simulink model "Autopilot_q_full_5may_new"  (R2020a)
settings: Solver=ode4  StartTime=0.0  StopTime=300  FixedStep=0.01  RelTol=1e-3
undefined symbols (not defined in the file or in its folder): Aero_cofficients, Atmosphere_pert, Atmospheric_model, Counter_sensor_model, Earth, error_global, flags_global, Guidance_Flags_global, INT_global, param_guidance, Payload_data, Plane_state_mode_finish_catcher_ftr_mode, Plane_state_mode_finish_catcher_fw_mode, Plane_state_mode_finish_catcher_q_mode, Plane_state_mode_finish_catcher_rtr_mode, Plane_state_store, propulsion_model, propulsion_model_int, Structural_data, Thrust_data_store, time_global, WGS84, Wind_data, Wind_model_int, Wind_pert_factor
libraries: simulink x33, aerolibactuator x15, cstblocks x3, aerolibatmos2 x2, aerolibfltsims x1, aerolibtransform2 x1, shared6dof x1
(part 6 of 10)

== system Autopilot_q_full_5may_new/AUTOPILOT /Autopilot Transition mode/Reverse transition/Pitch Controller/alpha controller ==
  acc_d : Inport
  Plane_state : Inport  Port=2
  Action Port : ActionPort  ActionPortLabel=else { }
  Aero_coffecients read2 : DataStoreRead  DataStoreName=Aero_cofficients  DataStoreElements=Aero_cofficients(:,:)
  Constant{6..11} (6 alike) : Constant
  Data Store Read : DataStoreRead  DataStoreName=Thrust_data_store  DataStoreElements=Thrust_data_store(:,:)
  Data Store Read1 : DataStoreRead  DataStoreName=Wind_data  DataStoreElements=Wind_data(:)
  Data Store Read13 : DataStoreRead  DataStoreName=propulsion_model  DataStoreElements=propulsion_model(:)
  Data Store Read15 : DataStoreRead  DataStoreName=Atmospheric_model
  Gain : Gain  Gain=57.3
  Gain1 : Gain  Gain=57.3
  MATLAB Function3 : MATLAB Function  TreatAsAtomicUnit=on
  PID Controller (2DOF)2 : simulink/Continuous/PID Controller (2DOF)  Controller=PID  TimeDomain=Discrete-time  SampleTime=0.01  IntegratorMethod=Forward Euler  FilterMethod=Forward Euler  Form=Parallel  UseFilter=on  ControllerParametersSource=internal  P=4.0  I=0.3  D=0.0  N=100  b=1  c=1  InitialConditionSource=internal  InitialConditionForIntegrator=0  InitialConditionForFilter=0  ExternalReset=none  ZeroCross=off  LimitOutput=off  UpperSaturationLimit=inf  LowerSaturationLimit=-inf  LinearizeAsGain=on  AntiWindupMode=none  Kb=1  TrackingMode=off  Kt=1  PParamMin=[]  PParamMax=[]  IParamMin=[]  IParamMax=[]  DParamMin=[]  DParamMax=[]  NParamMin=[]  NParamMax=[]  bParamMin=[]  bParamMax=[]  cParamMin=[]  cParamMax=[]  KbParamMin=[]  KbParamMax=[]  KtParamMin=[]  KtParamMax=[]  POutMin=[]  POutMax=[]  IOutMin=[]  IOutMax=[]  DOutMin=[]  DOutMax=[]  NOutMin=[]  NOutMax=[]  bOutMin=[]  bOutMax=[]  cOutMin=[]  cOutMax=[]  KbOutMin=[]  KbOutMax=[]  KtOutMin=[]  KtOutMax=[]  IntegratorOutMin=[]  IntegratorOutMax=[]  FilterOutMin=[]  FilterOutMax=[]  SumOutMin=[]  SumOutMax=[]  Sum1OutMin=[]  Sum1OutMax=[]  Sum2OutMin=[]  Sum2OutMax=[]  Sum3OutMin=[]  Sum3OutMax=[]  SumI1OutMin=[]  SumI1OutMax=[]  SumI2OutMin=[]  SumI2OutMax=[]  SumI3OutMin=[]  SumI3OutMax=[]  SumDOutMin=[]  SumDOutMax=[]  SaturationOutMin=[]  SaturationOutMax=[]  IntegratorContinuousStateAttributes=''  IntegratorStateMustResolveToSignalObject=off  IntegratorRTWStateStorageClass=Auto  FilterContinuousStateAttributes=''  FilterStateMustResolveToSignalObject=off  FilterRTWStateStorageClass=Auto  DifferentiatorICPrevScaledInput=0  DifferentiatorOutMin=[]  DifferentiatorOutMax=[]  FilterDiffOutCoefMin=[]  FilterDiffOutCoefMax=[]  SumDenOutMin=[]  SumDenOutMax=[]  SumNumOutMin=[]  SumNumOutMax=[]  ReciprocalOutMin=[]  ReciprocalOutMax=[]  DivideOutMin=[]  DivideOutMax=[]  TunerSelectOption=Transfer Function Based (PID Tuner App)
  Scope : Scope  NumInputPorts=2
  Structure_data_read1 : DataStoreRead  DataStoreName=Structural_data  DataStoreElements=Structural_data(:,:)
  alpha : Trigonometry  Operator=atan2
  u : DataStoreRead  DataStoreName=Plane_state_store  DataStoreElements=Plane_state_store(1,1)
  w : DataStoreRead  DataStoreName=Plane_state_store  DataStoreElements=Plane_state_store(1,3)
  Output : Outport  VectorParamsAs1DForOutWhenUnconnected=off
  wires:
  PID Controller (2DOF)2/1 -> Output/1
  Plane_state/1 -> MATLAB Function3/2(Plane_state)
  acc_d/1 -> MATLAB Function3/1(acc_d)
  MATLAB Function3/1(alpha_d) -> Gain/1, PID Controller (2DOF)2/1
  w/1 -> alpha/1
  u/1 -> alpha/2
  alpha/1 -> Gain1/1, PID Controller (2DOF)2/2
  Data Store Read/1 -> MATLAB Function3/5(Thrust)
  Aero_coffecients read2/1 -> MATLAB Function3/3(aero_data)
  Structure_data_read1/1 -> MATLAB Function3/4(structure_data)
  Gain1/1 -> Scope/2
  Gain/1 -> Scope/1
  Data Store Read1/1 -> MATLAB Function3/6(Wind_ned)
  Data Store Read13/1 -> MATLAB Function3/7(propulsion_data)
  Data Store Read15/1 -> MATLAB Function3/8(atmos_data)
  Constant6/1 -> MATLAB Function3/9(data2)
  Constant7/1 -> MATLAB Function3/10(data3)
  Constant8/1 -> MATLAB Function3/11(data4)
  Constant9/1 -> MATLAB Function3/12(data5)
  Constant10/1 -> MATLAB Function3/13(data6)
  Constant11/1 -> MATLAB Function3/14(data7)

== system Autopilot_q_full_5may_new/AUTOPILOT /Autopilot Transition mode/Reverse transition/Pitch Controller/theta controller ==
  time : Inport
  a_x_d : Inport  Port=2
  alpha_trim : Inport  Port=3
  Action Port : ActionPort  ActionPortLabel=if { }
  Data Store Read1 : DataStoreRead  DataStoreName=Thrust_data_store  DataStoreElements=Thrust_data_store(1,1:8)
  Gain : Gain  Gain=57.3
  Gain1 : Gain  Gain=57.3
  MATLAB Function3 : MATLAB Function  TreatAsAtomicUnit=on
  PID Controller (2DOF)2 : simulink/Continuous/PID Controller (2DOF)  Controller=PID  TimeDomain=Discrete-time  SampleTime=0.01  IntegratorMethod=Forward Euler  FilterMethod=Forward Euler  Form=Parallel  UseFilter=on  ControllerParametersSource=internal  P=2.0  I=0.0  D=0  N=100  b=1  c=1  InitialConditionSource=internal  InitialConditionForIntegrator=0  InitialConditionForFilter=0  ExternalReset=none  LimitOutput=off  UpperSaturationLimit=inf  LowerSaturationLimit=-inf  LinearizeAsGain=on  AntiWindupMode=none  Kb=1  TrackingMode=off  Kt=1  PParamMin=[]  PParamMax=[]  IParamMin=[]  IParamMax=[]  DParamMin=[]  DParamMax=[]  NParamMin=[]  NParamMax=[]  bParamMin=[]  bParamMax=[]  cParamMin=[]  cParamMax=[]  KbParamMin=[]  KbParamMax=[]  KtParamMin=[]  KtParamMax=[]  POutMin=[]  POutMax=[]  IOutMin=[]  IOutMax=[]  DOutMin=[]  DOutMax=[]  NOutMin=[]  NOutMax=[]  bOutMin=[]  bOutMax=[]  cOutMin=[]  cOutMax=[]  KbOutMin=[]  KbOutMax=[]  KtOutMin=[]  KtOutMax=[]  IntegratorOutMin=[]  IntegratorOutMax=[]  FilterOutMin=[]  FilterOutMax=[]  SumOutMin=[]  SumOutMax=[]  Sum1OutMin=[]  Sum1OutMax=[]  Sum2OutMin=[]  Sum2OutMax=[]  Sum3OutMin=[]  Sum3OutMax=[]  SumI1OutMin=[]  SumI1OutMax=[]  SumI2OutMin=[]  SumI2OutMax=[]  SumI3OutMin=[]  SumI3OutMax=[]  SumDOutMin=[]  SumDOutMax=[]  SaturationOutMin=[]  SaturationOutMax=[]  IntegratorContinuousStateAttributes=''  IntegratorStateMustResolveToSignalObject=off  IntegratorRTWStateStorageClass=Auto  FilterContinuousStateAttributes=''  FilterStateMustResolveToSignalObject=off  FilterRTWStateStorageClass=Auto  DifferentiatorICPrevScaledInput=0  DifferentiatorOutMin=[]  DifferentiatorOutMax=[]  FilterDiffOutCoefMin=[]  FilterDiffOutCoefMax=[]  SumDenOutMin=[]  SumDenOutMax=[]  SumNumOutMin=[]  SumNumOutMax=[]  ReciprocalOutMin=[]  ReciprocalOutMax=[]  DivideOutMin=[]  DivideOutMax=[]  TunerSelectOption=Transfer Function Based (PID Tuner App)
  Scope : Scope  NumInputPorts=2
  mass : DataStoreRead  DataStoreName=Structural_data  DataStoreElements=Structural_data(1,1)
  theta : DataStoreRead  DataStoreName=Plane_state_store  DataStoreElements=Plane_state_store(1,8)
  theta_dot : Outport  VectorParamsAs1DForOutWhenUnconnected=off
  wires:
  theta/1 -> PID Controller (2DOF)2/2, Gain1/1
  time/1 -> MATLAB Function3/1(t)
  Data Store Read1/1 -> MATLAB Function3/2(TT)
  a_x_d/1 -> MATLAB Function3/4(a_x_d)
  PID Controller (2DOF)2/1 -> theta_dot/1
  alpha_trim/1 -> MATLAB Function3/5(data)
  mass/1 -> MATLAB Function3/3(mass)
  MATLAB Function3/1(theta_d) -> Gain/1, PID Controller (2DOF)2/1
  Gain1/1 -> Scope/2
  Gain/1 -> Scope/1

== system Autopilot_q_full_5may_new/INITIALISE_PARAMS/If Action Subsystem/Aero_data_perturbation/Subsystem1/Subsystem ==
  CL_alpha : Constant
  CL_beta : Constant
  CL_delta_a : Constant
  CL_delta_e : Constant
  CL_delta_r : Constant
  CLo : Constant
  CLp : Constant
  CLq : Constant
  CLr : Constant
  Mux : Mux  Inputs=9
  Out1 : Outport  VectorParamsAs1DForOutWhenUnconnected=off
  wires:
  CL_delta_e/1 -> Mux/4
  CL_delta_r/1 -> Mux/6
  CLp/1 -> Mux/7
  CLo/1 -> Mux/1
  CL_alpha/1 -> Mux/2
  CLr/1 -> Mux/9
  CL_delta_a/1 -> Mux/5
  CL_beta/1 -> Mux/3
  CLq/1 -> Mux/8
  Mux/1 -> Out1/1

== system Autopilot_q_full_5may_new/INITIALISE_PARAMS/If Action Subsystem/Aero_data_perturbation/Subsystem2/Subsystem ==
  CL_alpha : Constant
  CL_beta : Constant
  CL_delta_a : Constant
  CL_delta_e : Constant
  CL_delta_r : Constant
  CLo : Constant
  CLp : Constant
  CLq : Constant
  CLr : Constant
  Mux : Mux  Inputs=9
  Out1 : Outport  VectorParamsAs1DForOutWhenUnconnected=off
  wires:
  Mux/1 -> Out1/1
  CLq/1 -> Mux/8
  CL_beta/1 -> Mux/3
  CL_delta_a/1 -> Mux/5
  CLr/1 -> Mux/9
  CL_alpha/1 -> Mux/2
  CLo/1 -> Mux/1
  CLp/1 -> Mux/7
  CL_delta_r/1 -> Mux/6
  CL_delta_e/1 -> Mux/4

== system Autopilot_q_full_5may_new/INITIALISE_PARAMS/If Action Subsystem/Aero_data_perturbation/Subsystem3/Subsystem ==
  CL_alpha : Constant
  CL_beta : Constant
  CL_delta_a : Constant
  CL_delta_e : Constant
  CL_delta_r : Constant
  CLo : Constant
  CLp : Constant
  CLq : Constant
  CLr : Constant
  Mux : Mux  Inputs=9
  Out1 : Outport  VectorParamsAs1DForOutWhenUnconnected=off
  wires:
  CL_delta_e/1 -> Mux/4
  CL_delta_r/1 -> Mux/6
  CLp/1 -> Mux/7
  CLo/1 -> Mux/1
  CL_alpha/1 -> Mux/2
  CLr/1 -> Mux/9
  CL_delta_a/1 -> Mux/5
  CL_beta/1 -> Mux/3
  CLq/1 -> Mux/8
  Mux/1 -> Out1/1

== system Autopilot_q_full_5may_new/INITIALISE_PARAMS/If Action Subsystem/Aero_data_perturbation/Subsystem4/Subsystem ==
  CL_alpha : Constant
  CL_beta : Constant
  CL_delta_a : Constant
  CL_delta_e : Constant
  CL_delta_r : Constant
  CLo : Constant
  CLp : Constant
  CLq : Constant
  CLr : Constant
  Mux : Mux  Inputs=9
  Out1 : Outport  VectorParamsAs1DForOutWhenUnconnected=off
  wires:
  Mux/1 -> Out1/1
  CLq/1 -> Mux/8
  CL_beta/1 -> Mux/3
  CL_delta_a/1 -> Mux/5
  CLr/1 -> Mux/9
  CL_alpha/1 -> Mux/2
  CLo/1 -> Mux/1
  CLp/1 -> Mux/7
  CL_delta_r/1 -> Mux/6
  CL_delta_e/1 -> Mux/4

== system Autopilot_q_full_5may_new/INITIALISE_PARAMS/If Action Subsystem/Aero_data_perturbation/Subsystem5/Subsystem ==
  CL_alpha : Constant
  CL_beta : Constant
  CL_delta_a : Constant
  CL_delta_e : Constant
  CL_delta_r : Constant
  CLo : Constant
  CLp : Constant
  CLq : Constant
  CLr : Constant
  Mux : Mux  Inputs=9
  Out1 : Outport  VectorParamsAs1DForOutWhenUnconnected=off
  wires:
  CL_delta_e/1 -> Mux/4
  CL_delta_r/1 -> Mux/6
  CLp/1 -> Mux/7
  CLo/1 -> Mux/1
  CL_alpha/1 -> Mux/2
  CLr/1 -> Mux/9
  CL_delta_a/1 -> Mux/5
  CL_beta/1 -> Mux/3
  CLq/1 -> Mux/8
  Mux/1 -> Out1/1

== system Autopilot_q_full_5may_new/INITIALISE_PARAMS/If Action Subsystem/Aero_data_perturbation/Subsystem6/Subsystem ==
  CL_alpha : Constant
  CL_beta : Constant
  CL_delta_a : Constant
  CL_delta_e : Constant
  CL_delta_r : Constant
  CLo : Constant
  CLp : Constant
  CLq : Constant
  CLr : Constant
  Mux : Mux  Inputs=9
  Out1 : Outport  VectorParamsAs1DForOutWhenUnconnected=off
  wires:
  Mux/1 -> Out1/1
  CLq/1 -> Mux/8
  CL_beta/1 -> Mux/3
  CL_delta_a/1 -> Mux/5
  CLr/1 -> Mux/9
  CL_alpha/1 -> Mux/2
  CLo/1 -> Mux/1
  CLp/1 -> Mux/7
  CL_delta_r/1 -> Mux/6
  CL_delta_e/1 -> Mux/4

== system Autopilot_q_full_5may_new/INITIALISE_PARAMS/If Action Subsystem/Atmosphere_pert/Subsystem1/Subsystem ==
  note: p
  note: density
  note: Temp
  note: a
  Constant{,1..3} (4 alike) : Constant
  Mux : Mux
  Out1 : Outport  VectorParamsAs1DForOutWhenUnconnected=off
  wires:
  Constant2/1 -> Mux/3
  Constant1/1 -> Mux/2
  Constant/1 -> Mux/1
  Constant3/1 -> Mux/4
  Mux/1 -> Out1/1

== system Autopilot_q_full_5may_new/INITIALISE_PARAMS/If Action Subsystem/Propulsion_data_pert/Subsystem1/Subsystem ==
  note: d_vtol
  note: b_vtol
  Constant : Constant
  Constant1 : Constant
  Mux : Mux  Inputs=2
  Out1 : Outport  VectorParamsAs1DForOutWhenUnconnected=off
  wires:
  Constant1/1 -> Mux/2
  Mux/1 -> Out1/1
  Constant/1 -> Mux/1

== system Autopilot_q_full_5may_new/INITIALISE_PARAMS/If Action Subsystem/Propulsion_data_pert/Subsystem2/Subsystem ==
  note: d_pusher
  note: b_pusher
  Constant2 : Constant
  Constant3 : Constant
  Mux1 : Mux  Inputs=2
  Out1 : Outport  VectorParamsAs1DForOutWhenUnconnected=off
  wires:
  Mux1/1 -> Out1/1
  Constant3/1 -> Mux1/2
  Constant2/1 -> Mux1/1

== system Autopilot_q_full_5may_new/INITIALISE_PARAMS/If Action Subsystem/Structure_data_pert/Subsystem1/Subsystem ==
  Constant : Constant
  Out1 : Outport  VectorParamsAs1DForOutWhenUnconnected=off
  wires:
  Constant/1 -> Out1/1

== system Autopilot_q_full_5may_new/INITIALISE_PARAMS/If Action Subsystem/Structure_data_pert/Subsystem2/Subsystem ==
  Constant : Constant
  Constant1 : Constant
  Constant2 : Constant
  Mux : Mux  Inputs=3
  Out1 : Outport  VectorParamsAs1DForOutWhenUnconnected=off
  wires:
  Constant/1 -> Mux/1
  Mux/1 -> Out1/1
  Constant1/1 -> Mux/2
  Constant2/1 -> Mux/3

== system Autopilot_q_full_5may_new/INITIALISE_PARAMS/If Action Subsystem/Structure_data_pert/Subsystem3/Subsystem ==
  Constant{3..8} (6 alike) : Constant
  Mux1 : Mux  Inputs=6
  Out1 : Outport  VectorParamsAs1DForOutWhenUnconnected=off
  wires:
  Constant8/1 -> Mux1/6
  Mux1/1 -> Out1/1
  Constant3/1 -> Mux1/1
  Constant7/1 -> Mux1/5
  Constant5/1 -> Mux1/3
  Constant4/1 -> Mux1/2
  Constant6/1 -> Mux1/4

== system Autopilot_q_full_5may_new/INITIALISE_PARAMS/If Action Subsystem/Structure_data_pert/Subsystem4/Subsystem ==
  note: y9
  note: z1
  note: y10
  note: y5
  note: y7
  note: y6
  note: x2 y
  note: y2
  note: x1
  note: y8
  note: y4
  note: y1
  note: y3
  Constant{9..21} (13 alike) : Constant
  Mux2 : Mux  Inputs=13
  Out1 : Outport  VectorParamsAs1DForOutWhenUnconnected=off
  wires:
  Constant20/1 -> Mux2/7
  Constant17/1 -> Mux2/10
  Constant15/1 -> Mux2/8
  Constant19/1 -> Mux2/12
  Constant21/1 -> Mux2/13
  Constant12/1 -> Mux2/4
  Constant11/1 -> Mux2/3
  Mux2/1 -> Out1/1
  Constant10/1 -> Mux2/2
  Constant18/1 -> Mux2/11
  Constant14/1 -> Mux2/6
  Constant13/1 -> Mux2/5
  Constant16/1 -> Mux2/9
  Constant9/1 -> Mux2/1

== system Autopilot_q_full_5may_new/INITIALISE_PARAMS/If Action Subsystem/Structure_data_pert/Subsystem5/Subsystem ==
  mb_pert : Constant
  Out1 : Outport  VectorParamsAs1DForOutWhenUnconnected=off
  wires:
  mb_pert/1 -> Out1/1

== system Autopilot_q_full_5may_new/INITIALISE_PARAMS/If Action Subsystem/Wind_data_pert/Subsystem1/Subsystem ==
  note: V_N
  note: V_D
  note: V_E
  Constant : Constant
  Constant1 : Constant
  Constant2 : Constant
  Mux : Mux  Inputs=3
  Out1 : Outport  VectorParamsAs1DForOutWhenUnconnected=off
  wires:
  Constant/1 -> Mux/1
  Mux/1 -> Out1/1
  Constant1/1 -> Mux/2
  Constant2/1 -> Mux/3

== matlab function Autopilot_q_full_5may_new/All SENSOR MODEL2/MATLAB Function1 ==
  settings: updateMethod=DISCRETE
  data: sigma input; mu input; y output
function y = fcn(sigma,mu)
y=normrnd(mu,sigma);
end

== matlab function Autopilot_q_full_5may_new/All SENSOR MODEL2/MATLAB Function10 ==
  settings: updateMethod=DISCRETE
  data: sigma input; mu input; y output
function y = fcn(sigma,mu)
y=normrnd(mu,sigma);
end

== matlab function Autopilot_q_full_5may_new/All SENSOR MODEL2/MATLAB Function11 ==
  settings: updateMethod=DISCRETE
  data: sigma input; mu input; y output
function y = fcn(sigma,mu)
y=normrnd(mu,sigma);
end

== matlab function Autopilot_q_full_5may_new/All SENSOR MODEL2/MATLAB Function2 ==
  data: sigma input; mu input; y output
function y = fcn(sigma,mu)
y=normrnd(mu,sigma);
end

== matlab function Autopilot_q_full_5may_new/All SENSOR MODEL2/MATLAB Function3 ==
  data: sigma input; mu input; y output
function y = fcn(sigma,mu)
y=normrnd(mu,sigma);
end

== matlab function Autopilot_q_full_5may_new/All SENSOR MODEL2/MATLAB Function4 ==
  data: sigma input; mu input; y output
function y = fcn(sigma,mu)
y=normrnd(mu,sigma);
end

== matlab function Autopilot_q_full_5may_new/All SENSOR MODEL2/MATLAB Function5 ==
  data: sigma input; mu input; y output
function y = fcn(sigma,mu)
y=normrnd(mu,sigma);
end

== matlab function Autopilot_q_full_5may_new/All SENSOR MODEL2/MATLAB Function6 ==
  data: sigma input; mu input; y output
function y = fcn(sigma,mu)
y=normrnd(mu,sigma);
end

== matlab function Autopilot_q_full_5may_new/All SENSOR MODEL2/MATLAB Function7 ==
  data: sigma input; mu input; y output
function y = fcn(sigma,mu)
y=normrnd(mu,sigma);
end

== matlab function Autopilot_q_full_5may_new/All SENSOR MODEL2/MATLAB Function8 ==
  data: sigma input; mu input; y output
function y = fcn(sigma,mu)
y=normrnd(mu,sigma);
end

== matlab function Autopilot_q_full_5may_new/AUTOPILOT /Autopilot Transition mode/Reverse transition/Pitch Controller/MATLAB Function ==
  data: u1 input; u2 input; y output
function y = fcn(u1, u2)

if u1<u2    
    y=1; 
else
    y=0;
end


end

== matlab function Autopilot_q_full_5may_new/Wind_Model/Subsystem2/MATLAB Function ==
  data: u input; y output; Wind_model_int input; Z input
function y = fcn(u, Wind_model_int, Z)
y=u;
turb_50=Wind_model_int(8);
turb_50_600=Wind_model_int(9);
turb_600=Wind_model_int(10);

if ((turb_50 == 0) && (Z >=-50))
    y=0.0;  
end

if ((turb_50_600 == 0) && (Z >=-600) && (Z <=-50))
    y=0.0;  
end

if ((turb_600 == 0) && (Z <=-600))
    y=0.0;  
end

if Z>0.0
    y=0.0;
end
end

== matlab function Autopilot_q_full_5may_new/Forces and moments/Forces and moments ==
  data: Tzf1 input; Tzf2 input; Tzf3 input; Tzf4 input; Tzb5 input; Tzb6 input; Tzb7 input; Tzb8 input; Tx9 input; Tx10 input; delta_e input; delta_a input; delta_r input; fx output; fy output; fz output; l output; m output; n output; aero_data input; structure_data input; ideal_Plane_state input; Payload_f_m input; Wind_ned input; flags_global input; propulsion_data input; atmos_data input; wind_pert_factor input; propulsion_pert_factor input; structure_pert_factor input; atmos_pert_factor input; aero_coff_pert_factor input; data7 input; data8 input; data9 input; data10 input; data11 input; data12 input
function [fx,fy,fz,l,m,n] = fcn(Tzf1,Tzf2,Tzf3,Tzf4,Tzb5,Tzb6,Tzb7,Tzb8,Tx9,Tx10,delta_e,delta_a,delta_r, aero_data,structure_data , ideal_Plane_state, Payload_f_m,Wind_ned, flags_global, propulsion_data, atmos_data, wind_pert_factor, propulsion_pert_factor, structure_pert_factor, atmos_pert_factor, aero_coff_pert_factor, data7, data8, data9, data10, data11, data12)


quad_mode=flags_global(3);
Transition_mode=flags_global(4);
Fixed_wing_mode=flags_global(5);

%%
b1=propulsion_data(1); % b and d of vtol propellers
d1=propulsion_data(2);

b1 = b1*propulsion_pert_factor(1); % adding in perturbation in b and d
d1 = d1*propulsion_pert_factor(2);
b1_inv=1.0/b1;
%%
rho=atmos_data(4); % density
rho = rho*atmos_pert_factor(4); % adding perturbation in density
%%
mass=structure_data(1,1);c=structure_data(1,2);b=structure_data(1,3);s=structure_data(1,4);
Ix=structure_data(1,5);Iy=structure_data(1,6);Iz=structure_data(1,7);
Ixy=structure_data(1,8);Ixz=structure_data(1,9);Iyz=structure_data(1,10);
x1=structure_data(1,11);x2=structure_data(1,12);y1=structure_data(1,13);y2=structure_data(1,14);
y3=structure_data(1,15);y4=structure_data(1,16);y5=structure_data(1,17);y6=structure_data(1,18);
y7=structure_data(1,19);y8=structure_data(1,20);y9=structure_data(1,21);y10=structure_data(1,22);
z9=structure_data(1,23);mb=structure_data(1,24);
%%
mass=mass*structure_pert_factor(1,1); % perturbation in structure data
c=c*structure_pert_factor(1,2);b=b*structure_pert_factor(1,3);s=s*structure_pert_factor(1,4);
Ix=Ix*structure_pert_factor(1,5);Iy=Iy*structure_pert_factor(1,6);Iz=Iz*structure_pert_factor(1,7);
Ixy=Ixy*structure_pert_factor(1,8);Ixz=Ixz*structure_pert_factor(1,9);Iyz=Iyz*structure_pert_factor(1,10);
x1=x1*structure_pert_factor(1,11);x2=x2*structure_pert_factor(1,12);
y1=y1*structure_pert_factor(1,13);y2=y2*structure_pert_factor(1,14);y3=y3*structure_pert_factor(1,15);y4=y4*structure_pert_factor(1,16);
y5=y5*structure_pert_factor(1,17);y6=y6*structure_pert_factor(1,18);y7=y7*structure_pert_factor(1,19);y8=y8*structure_pert_factor(1,20);
y9=y9*structure_pert_factor(1,21);y10=y10*structure_pert_factor(1,22);
z9=z9*structure_pert_factor(1,23);
mb=mb*structure_pert_factor(1,24);
z10=-z9;
%%
c0=Ix*Iz-Ixz^2;
c1=Ixz*(Ix-Iy+Iz)/c0;
c2=(Iz*(Iz-Iy)+Ixz^2)/c0;
c3=Iz/c0;
c4=Ixz/c0;
c5=(Iz-Ix)/c0;
c6=Ixz/Iy;
c7=((Ix-Iy)*Ix + Ixz^2)/c0;
c8=Ix/c0;
%%

CLo =aero_data(1,1); CL_alpha=aero_data(1,2);CL_beta=aero_data(1,3); CL_delta_e=aero_data(1,4); CL_delta_a=aero_data(1,5); CL_delta_r=aero_data(1,6); CL_p=aero_data(1,7);CL_q=aero_data(1,8);CL_r=aero_data(1,9);

Cdo =aero_data(2,1); Cd_alpha=aero_data(2,2);Cd_beta=aero_data(2,3); Cd_delta_e=aero_data(2,4); Cd_delta_a=aero_data(2,5); Cd_delta_r=aero_data(2,6); Cd_p=aero_data(2,7);Cd_q=aero_data(2,8);Cd_r=aero_data(2,9);

CYo =aero_data(3,1); CY_alpha=aero_data(3,2);CY_beta=aero_data(3,3); CY_delta_e=aero_data(3,4); CY_delta_a=aero_data(3,5); CY_delta_r=aero_data(3,6); CY_p=aero_data(3,7);CY_q=aero_data(3,8);CY_r=aero_data(3,9);

Clo =aero_data(4,1); Cl_alpha=aero_data(4,2);Cl_beta=aero_data(4,3); Cl_delta_e=aero_data(4,4); Cl_delta_a=aero_data(4,5); Cl_delta_r=aero_data(4,6); Cl_p=aero_data(4,7);Cl_q=aero_data(4,8);Cl_r=aero_data(4,9);

Cmo =aero_data(5,1); Cm_alpha=aero_data(5,2);Cm_beta=aero_data(5,3); Cm_delta_e=aero_data(5,4); Cm_delta_a=aero_data(5,5); Cm_delta_r=aero_data(5,6); Cm_p=aero_data(5,7);Cm_q=aero_data(5,8);Cm_r=aero_data(5,9);

Cno =aero_data(6,1); Cn_alpha=aero_data(6,2);Cn_beta=aero_data(6,3); Cn_delta_e=aero_data(6,4); Cn_delta_a=aero_data(6,5); Cn_delta_r=aero_data(6,6); Cn_p=aero_data(6,7);Cn_q=aero_data(6,8);Cn_r=aero_data(6,9);

if quad_mode ==1
    aero_data(:,:)=0.0;
    CLo =aero_data(1,1); CL_alpha=aero_data(1,2);CL_beta=aero_data(1,3); CL_delta_e=aero_data(1,4); CL_delta_a=aero_data(1,5); CL_delta_r=aero_data(1,6); CL_p=aero_data(1,7);CL_q=aero_data(1,8);CL_r=aero_data(1,9);
    
    Cdo =aero_data(2,1); Cd_alpha=aero_data(2,2);Cd_beta=aero_data(2,3); Cd_delta_e=aero_data(2,4); Cd_delta_a=aero_data(2,5); Cd_delta_r=aero_data(2,6); Cd_p=aero_data(2,7);Cd_q=aero_data(2,8);Cd_r=aero_data(2,9);
    
    CYo =aero_data(3,1); CY_alpha=aero_data(3,2);CY_beta=aero_data(3,3); CY_delta_e=aero_data(3,4); CY_delta_a=aero_data(3,5); CY_delta_r=aero_data(3,6); CY_p=aero_data(3,7);CY_q=aero_data(3,8);CY_r=aero_data(3,9);
    
    Clo =aero_data(4,1); Cl_alpha=aero_data(4,2);Cl_beta=aero_data(4,3); Cl_delta_e=aero_data(4,4); Cl_delta_a=aero_data(4,5); Cl_delta_r=aero_data(4,6); Cl_p=aero_data(4,7);Cl_q=aero_data(4,8);Cl_r=aero_data(4,9);
    
    Cmo =aero_data(5,1); Cm_alpha=aero_data(5,2);Cm_beta=aero_data(5,3); Cm_delta_e=aero_data(5,4); Cm_delta_a=aero_data(5,5); Cm_delta_r=aero_data(5,6); Cm_p=aero_data(5,7);Cm_q=aero_data(5,8);Cm_r=aero_data(5,9);
    
    Cno =aero_data(6,1); Cn_alpha=aero_data(6,2);Cn_beta=aero_data(6,3); Cn_delta_e=aero_data(6,4); Cn_delta_a=aero_data(6,5); Cn_delta_r=aero_data(6,6); Cn_p=aero_data(6,7);Cn_q=aero_data(6,8);Cn_r=aero_data(6,9);
end

if Fixed_wing_mode ==1
    
    CLo =aero_data(1,1); CL_alpha=aero_data(1,2);CL_beta=aero_data(1,3); CL_delta_e=aero_data(1,4); CL_delta_a=aero_data(1,5); CL_delta_r=aero_data(1,6); CL_p=aero_data(1,7);CL_q=aero_data(1,8);CL_r=aero_data(1,9);
    
    Cdo =aero_data(2,1); Cd_alpha=aero_data(2,2);Cd_beta=aero_data(2,3); Cd_delta_e=aero_data(2,4); Cd_delta_a=aero_data(2,5); Cd_delta_r=aero_data(2,6); Cd_p=aero_data(2,7);Cd_q=aero_data(2,8);Cd_r=aero_data(2,9);
    
    CYo =aero_data(3,1); CY_alpha=aero_data(3,2);CY_beta=aero_data(3,3); CY_delta_e=aero_data(3,4); CY_delta_a=aero_data(3,5); CY_delta_r=aero_data(3,6); CY_p=aero_data(3,7);CY_q=aero_data(3,8);CY_r=aero_data(3,9);
    
    Clo =aero_data(4,1); Cl_alpha=aero_data(4,2);Cl_beta=aero_data(4,3); Cl_delta_e=aero_data(4,4); Cl_delta_a=aero_data(4,5); Cl_delta_r=aero_data(4,6); Cl_p=aero_data(4,7);Cl_q=aero_data(4,8);Cl_r=aero_data(4,9);
    
    Cmo =aero_data(5,1); Cm_alpha=aero_data(5,2);Cm_beta=aero_data(5,3); Cm_delta_e=aero_data(5,4); Cm_delta_a=aero_data(5,5); Cm_delta_r=aero_data(5,6); Cm_p=aero_data(5,7);Cm_q=aero_data(5,8);Cm_r=aero_data(5,9);
    
    Cno =aero_data(6,1); Cn_alpha=aero_data(6,2);Cn_beta=aero_data(6,3); Cn_delta_e=aero_data(6,4); Cn_delta_a=aero_data(6,5); Cn_delta_r=aero_data(6,6); Cn_p=aero_data(6,7);Cn_q=aero_data(6,8);Cn_r=aero_data(6,9);
end

if Transition_mode==1
    CLo =aero_data(1,1); CL_alpha=aero_data(1,2);CL_beta=aero_data(1,3); CL_delta_e=aero_data(1,4); CL_delta_a=aero_data(1,5); CL_delta_r=aero_data(1,6); CL_p=aero_data(1,7);CL_q=aero_data(1,8);CL_r=aero_data(1,9);
    
    Cdo =aero_data(2,1); Cd_alpha=aero_data(2,2);Cd_beta=aero_data(2,3); Cd_delta_e=aero_data(2,4); Cd_delta_a=aero_data(2,5); Cd_delta_r=aero_data(2,6); Cd_p=aero_data(2,7);Cd_q=aero_data(2,8);Cd_r=aero_data(2,9);
    
    CYo =aero_data(3,1); CY_alpha=aero_data(3,2);CY_beta=aero_data(3,3); CY_delta_e=aero_data(3,4); CY_delta_a=aero_data(3,5); CY_delta_r=aero_data(3,6); CY_p=aero_data(3,7);CY_q=aero_data(3,8);CY_r=aero_data(3,9);
    
    Clo =aero_data(4,1); Cl_alpha=aero_data(4,2);Cl_beta=aero_data(4,3); Cl_delta_e=aero_data(4,4); Cl_delta_a=aero_data(4,5); Cl_delta_r=aero_data(4,6); Cl_p=aero_data(4,7);Cl_q=aero_data(4,8);Cl_r=aero_data(4,9);
    
    Cmo =aero_data(5,1); Cm_alpha=aero_data(5,2);Cm_beta=aero_data(5,3); Cm_delta_e=aero_data(5,4); Cm_delta_a=aero_data(5,5); Cm_delta_r=aero_data(5,6); Cm_p=aero_data(5,7);Cm_q=aero_data(5,8);Cm_r=aero_data(5,9);
    
    Cno =aero_data(6,1); Cn_alpha=aero_data(6,2);Cn_beta=aero_data(6,3); Cn_delta_e=aero_data(6,4); Cn_delta_a=aero_data(6,5); Cn_delta_r=aero_data(6,6); Cn_p=aero_data(6,7);Cn_q=aero_data(6,8);Cn_r=aero_data(6,9);
end
%% perturbation in Aero coffecients
CLo =CLo*aero_coff_pert_factor(1,1); CL_alpha=CL_alpha*aero_coff_pert_factor(1,2);CL_beta=CL_beta*aero_coff_pert_factor(1,3); CL_delta_e=CL_delta_e*aero_coff_pert_factor(1,4); CL_delta_a=CL_delta_a*aero_coff_pert_factor(1,5); CL_delta_r=CL_delta_r*aero_coff_pert_factor(1,6); CL_p=CL_p*aero_coff_pert_factor(1,7);CL_q=CL_q*aero_coff_pert_factor(1,8);CL_r=CL_r*aero_coff_pert_factor(1,9);

Cdo =Cdo*aero_coff_pert_factor(2,1); Cd_alpha=Cd_alpha*aero_coff_pert_factor(2,2);Cd_beta=Cd_beta*aero_coff_pert_factor(2,3); Cd_delta_e=Cd_delta_e*aero_coff_pert_factor(2,4); Cd_delta_a=Cd_delta_a*aero_coff_pert_factor(2,5); Cd_delta_r=Cd_delta_r*aero_coff_pert_factor(2,6); Cd_p=Cd_p*aero_coff_pert_factor(2,7);Cd_q=Cd_q*aero_coff_pert_factor(2,8);Cd_r=Cd_r*aero_coff_pert_factor(2,9);

CYo =CYo*aero_coff_pert_factor(3,1); CY_alpha=CY_alpha*aero_coff_pert_factor(3,2);CY_beta=CY_beta*aero_coff_pert_factor(3,3); CY_delta_e=CY_delta_e*aero_coff_pert_factor(3,4); CY_delta_a=CY_delta_a*aero_coff_pert_factor(3,5); CY_delta_r=CY_delta_r*aero_coff_pert_factor(3,6); CY_p=CY_p*aero_coff_pert_factor(3,7);CY_q=CY_q*aero_coff_pert_factor(3,8);CY_r=CY_r*aero_coff_pert_factor(3,9);

Clo =Clo*aero_coff_pert_factor(4,1); Cl_alpha=Cl_alpha*aero_coff_pert_factor(4,2);Cl_beta=Cl_beta*aero_coff_pert_factor(4,3); Cl_delta_e=Cl_delta_e*aero_coff_pert_factor(4,4); Cl_delta_a=Cl_delta_a*aero_coff_pert_factor(4,5); Cl_delta_r=Cl_delta_r*aero_coff_pert_factor(4,6); Cl_p=Cl_p*aero_coff_pert_factor(4,7);Cl_q=Cl_q*aero_coff_pert_factor(4,8);Cl_r=Cl_r*aero_coff_pert_factor(4,9);

Cmo =Cmo*aero_coff_pert_factor(5,1); Cm_alpha=Cm_alpha*aero_coff_pert_factor(5,2);Cm_beta=Cm_beta*aero_coff_pert_factor(5,3); Cm_delta_e=Cm_delta_e*aero_coff_pert_factor(5,4); Cm_delta_a=Cm_delta_a*aero_coff_pert_factor(5,5); Cm_delta_r=Cm_delta_r*aero_coff_pert_factor(5,6); Cm_p=Cm_p*aero_coff_pert_factor(5,7);Cm_q=Cm_q*aero_coff_pert_factor(5,8);Cm_r=Cm_r*aero_coff_pert_factor(5,9);

Cno =Cno*aero_coff_pert_factor(6,1); Cn_alpha=Cn_alpha*aero_coff_pert_factor(6,2);Cn_beta=Cn_beta*aero_coff_pert_factor(6,3); Cn_delta_e=Cn_delta_e*aero_coff_pert_factor(6,4); Cn_delta_a=Cn_delta_a*aero_coff_pert_factor(6,5); Cn_delta_r=Cn_delta_r*aero_coff_pert_factor(6,6); Cn_p=Cn_p*aero_coff_pert_factor(6,7);Cn_q=Cn_q*aero_coff_pert_factor(6,8);Cn_r=Cn_r*aero_coff_pert_factor(6,9);
%%
Cd_brake=0.0;brake=0.0;g=9.81;
%%
u=ideal_Plane_state(1);
v=ideal_Plane_state(2);
w=ideal_Plane_state(3);
p=ideal_Plane_state(4);
q=ideal_Plane_state(5);
r=ideal_Plane_state(6);
phi=ideal_Plane_state(7);
theta=ideal_Plane_state(8);
psi=ideal_Plane_state(9);
X=ideal_Plane_state(10);
Y=ideal_Plane_state(11);
Z=ideal_Plane_state(12);
%%


Tzf=Tzf2+Tzf3;
Tzb=Tzb6+Tzb7;
%%

R_v_v1=[cos(psi) sin(psi) 0; -sin(psi) cos(psi) 0; 0 0 1];
R_v1_v2=[cos(theta) 0 -sin(theta) ;0 1 0; sin(theta) 0 cos(theta)];
R_v2_b=[1 0 0;0 cos(phi) sin(phi) ;0 -sin(phi) cos(phi)];
R_v_b=R_v2_b*R_v1_v2*R_v_v1;

%%

Wind_ned(1)=Wind_ned(1)*wind_pert_factor(1);% adding perturbation to wind components
Wind_ned(2)=Wind_ned(2)*wind_pert_factor(2);
Wind_ned(3)=Wind_ned(3)*wind_pert_factor(3);

V_wind_bd=R_v_b*[Wind_ned(1);Wind_ned(2);Wind_ned(3)];

ppp = [u-V_wind_bd(1); v-V_wind_bd(2); w-V_wind_bd(3)];
u_r=ppp(1);
v_r=ppp(2);
w_r=ppp(3);
V=sqrt(u_r^2+v_r^2+w_r^2);

%%

if (u_r^2+v_r^2+w_r^2)<=0.01
    alpha=0;
else
    alpha=atan2( w_r, u_r);
end


if norm(u_r) < 10^-3  && norm(v_r) < 10^-3 && norm(w_r) < 10^-3
    beta=0;
else
    beta = asin(v_r/sqrt(u_r^2+v_r^2+w_r^2));
end
%%


R_b_s=[cos(alpha) 0 sin(alpha) ;0 1 0; -sin(alpha) 0 cos(alpha)];
R_s_w=[cos(beta) sin(beta) 0; -sin(beta) cos(beta) 0; 0 0 1];
R_w_b=(R_b_s)'*(R_s_w)';

%%


mg_b = R_v_b*[0 ;0; mass*g];
D=0.5*rho*V*V*s*(Cdo+Cd_alpha*abs(alpha)+Cd_delta_e*abs(delta_e)+ Cd_brake*abs(brake)) ;
D_b=R_w_b*[-D;0;0];

if V<0.1
    CL = CLo + CL_alpha*alpha + CL_delta_e*delta_e ;
else
    CL = CLo + CL_alpha*alpha + CL_delta_e*delta_e  + CL_q*q*c/(2*V) ;
end
L=0.5*rho*V*V*s*(CL);
L_b = R_w_b*[0;0;-L];
if abs(V)<0.1
    CY=CYo + CY_delta_r*delta_r + CY_beta*beta;
else
    CY=CYo + CY_delta_r*delta_r + CY_beta*beta + CY_r*r*b/(2*V);
end
FY=0.5*rho*V*V*s*(CY);
%%

l_aero=0.5*rho*V^2*s*b*( Clo + Cl_delta_a*delta_a +Cl_delta_r*delta_r +Cl_beta*beta )+0.5*rho*V*s*b*(Cl_p*p*b/2+Cl_r*r*b/2);
m_aero=0.5*rho*V^2*s*c*( Cmo + Cm_alpha*alpha + Cm_delta_e*delta_e)+0.5*rho*V*s*c*Cm_q*q*c/2;
n_aero=0.5*rho*V^2*s*b*( Cno + Cn_delta_a*delta_a +Cn_delta_r*delta_r +Cn_beta*beta )+0.5*rho*V*s*b*(Cn_r*r*b/2+ Cn_p*p*b/2);


l=Payload_f_m(3) + l_aero - Tzf2*y2*cos(mb) - Tzf3*y3*cos(mb)   - Tzb6*y6*cos(mb) - Tzb7*y7*cos(mb);
m=Payload_f_m(4) + m_aero + Tzf*x1*cos(mb) + Tzb*x2*cos(mb) + Tx9*z9 + d1*Tzf2*b1_inv*sin(mb) - d1*Tzf3*b1_inv*sin(mb) - d1*Tzb6*b1_inv*sin(mb) + d1*Tzb7*b1_inv*sin(mb) ;
%n=n_aero - Tx9_real*y9  - d1*Tzf2_real/b1 + d1*Tzf3_real/b1 + d1*Tzb6_real/b1 - d1*Tzb7_real/b1 ; //optimization
n=Payload_f_m(5) + n_aero - Tx9*y9 - Tx10*y10 + (Tzf2*x1*sin(mb) - Tzf3*x1*sin(mb) +  Tzb6*x2*sin(mb) - Tzb7*x2*sin(mb)) - d1*Tzf2*b1_inv*cos(mb) + d1*Tzf3*b1_inv*cos(mb)  + d1*Tzb6*b1_inv*cos(mb)  - d1*Tzb7*b1_inv*cos(mb)  ;



fx = Payload_f_m(1) +  Tx9 + Tx10 + D_b(1)+ mg_b(1)+L_b(1);
%%%%%%%%%%%%%%%%%%%%%%%%%%%%%%%%%%%%%%%%%%%%%%%%%%%%%%%%%%%%%%%%%%%%%%%%%%%
fy = Payload_f_m(2) + (Tzf2*sin(mb) - Tzf3*sin(mb) + Tzb6*sin(mb) - Tzb7*sin(mb)) + D_b(2) + mg_b(2) + FY + L_b(2);
%%%%%%%%%%%%%%%%%%%%%%%%%%%%%%%%%%%%%%%%%%%%%%%%%%%%%%%%%%%%%%%%%%%%%%%%%%%
fz = Payload_f_m(3) -  Tzf*cos(mb) - Tzb*cos(mb) + mg_b(3)+D_b(3)+L_b(3);



end

== matlab function Autopilot_q_full_5may_new/All SENSOR MODEL2/MATLAB Function9 ==
  data: sigma input; mu input; y output
function y = fcn(sigma,mu)
y=normrnd(mu,sigma);
end

== matlab function Autopilot_q_full_5may_new/AUTOPILOT /Autopilot Quad mode/Autopilot ==
  data: q_dot_d input; p_dot_d input; r_dot_d input; acc_d input; Tzf1 output; Tzf2 output; Tzf3 output; Tzf4 output; Tzb5 output; Tzb6 output; Tzb7 output; Tzb8 output; Tx9 output; Tx10 output; delta_e output; delta_a output; delta_r output; Plane_state input; aero_data input; structure_data input; Thrust input; Wind_ned input; propulsion_data input; atmos_data input; wind_pert_factor input; propulsion_pert_factor input; structure_pert_factor input; atmos_pert_factor input; aero_coff_pert_factor input; data7 input; data8 input; data9 input; data10 input; data11 input; data12 input
function [Tzf1,Tzf2,Tzf3,Tzf4,Tzb5,Tzb6,Tzb7,Tzb8,Tx9,Tx10,delta_e,delta_a,delta_r]= Autopilot(q_dot_d,p_dot_d,r_dot_d,acc_d,Plane_state, aero_data, structure_data, Thrust, Wind_ned,propulsion_data, atmos_data, wind_pert_factor, propulsion_pert_factor, structure_pert_factor, atmos_pert_factor, aero_coff_pert_factor, data7, data8, data9, data10, data11, data12)


aero_data(:,:)=0.0;


b1=propulsion_data(1); % b and d of vtol propellers
d1=propulsion_data(2);
b1_inv=1.0/b1;
% b1 = b1*propulsion_pert_factor(1); % adding in perturbation in b and d
% d1 = d1*propulsion_pert_factor(2);
% b1_inv=1.0/b1;

rho=atmos_data(4); % density
%rho = rho*atmos_pert_factor(4); % adding perturbation in density

Tzf1=Thrust(1);
Tzf2=Thrust(2);
Tzf3=Thrust(3);
Tzf4=Thrust(4);

Tzb5=Thrust(5);
Tzb6=Thrust(6);
Tzb7=Thrust(7);
Tzb8=Thrust(8);
Tx9=Thrust(9);
Tx10=Thrust(10);
delta_e=Thrust(11);
delta_a=Thrust(12);
delta_r=Thrust(13);

%%
mass=structure_data(1,1);c=structure_data(1,2);b=structure_data(1,3);s=structure_data(1,4);
Ix=structure_data(1,5);Iy=structure_data(1,6);Iz=structure_data(1,7);
Ixy=structure_data(1,8);Ixz=structure_data(1,9);Iyz=structure_data(1,10);
x1=structure_data(1,11);x2=structure_data(1,12);y1=structure_data(1,13);y2=structure_data(1,14);
y3=structure_data(1,15);y4=structure_data(1,16);y5=structure_data(1,17);y6=structure_data(1,18);
y7=structure_data(1,19);y8=structure_data(1,20);y9=structure_data(1,21);y10=structure_data(1,22);
z9=structure_data(1,23);mb=structure_data(1,24);
%%
% mass=mass*structure_pert_factor(1,1); % perturbation in structure data
% c=c*structure_pert_factor(1,2);b=b*structure_pert_factor(1,3);s=s*structure_pert_factor(1,4);
% Ix=Ix*structure_pert_factor(1,5);Iy=Iy*structure_pert_factor(1,6);Iz=Iz*structure_pert_factor(1,7);
% Ixy=Ixy*structure_pert_factor(1,8);Ixz=Ixz*structure_pert_factor(1,9);Iyz=Iyz*structure_pert_factor(1,10);
% x1=x1*structure_pert_factor(1,11);x2=x2*structure_pert_factor(1,12);
% y1=y1*structure_pert_factor(1,13);y2=y2*structure_pert_factor(1,14);y3=y3*structure_pert_factor(1,15);y4=y4*structure_pert_factor(1,16);
% y5=y5*structure_pert_factor(1,17);y6=y6*structure_pert_factor(1,18);y7=y7*structure_pert_factor(1,19);y8=y8*structure_pert_factor(1,20);
% y9=y9*structure_pert_factor(1,21);y10=y10*structure_pert_factor(1,22);
% z9=z9*structure_pert_factor(1,23);
% mb=mb*structure_pert_factor(1,24);
%%
T_by_W=2.0;
%%
c0=Ix*Iz-Ixz^2;
c1=Ixz*(Ix-Iy+Iz)/c0;
c2=(Iz*(Iz-Iy)+Ixz^2)/c0;
c3=Iz/c0;
c4=Ixz/c0;
c5=(Iz-Ix)/c0;
c6=Ixz/Iy;
c7=((Ix-Iy)*Ix + Ixz^2)/c0;
c8=Ix/c0;
c3_inv=1/c3;
c8_inv=1/c8;
%%

CLo =aero_data(1,1); CL_alpha=aero_data(1,2);CL_beta=aero_data(1,3); CL_delta_e=aero_data(1,4); CL_delta_a=aero_data(1,5); CL_delta_r=aero_data(1,6); CL_p=aero_data(1,7);CL_q=aero_data(1,8);CL_r=aero_data(1,9);

Cdo =aero_data(2,1); Cd_alpha=aero_data(2,2);Cd_beta=aero_data(2,3); Cd_delta_e=aero_data(2,4); Cd_delta_a=aero_data(2,5); Cd_delta_r=aero_data(2,6); Cd_p=aero_data(2,7);Cd_q=aero_data(2,8);Cd_r=aero_data(2,9);

CYo =aero_data(3,1); CY_alpha=aero_data(3,2);CY_beta=aero_data(3,3); CY_delta_e=aero_data(3,4); CY_delta_a=aero_data(3,5); CY_delta_r=aero_data(3,6); CY_p=aero_data(3,7);CY_q=aero_data(3,8);CY_r=aero_data(3,9);

Clo =aero_data(4,1); Cl_alpha=aero_data(4,2);Cl_beta=aero_data(4,3); Cl_delta_e=aero_data(4,4); Cl_delta_a=aero_data(4,5); Cl_delta_r=aero_data(4,6); Cl_p=aero_data(4,7);Cl_q=aero_data(4,8);Cl_r=aero_data(4,9);

Cmo =aero_data(5,1); Cm_alpha=aero_data(5,2);Cm_beta=aero_data(5,3); Cm_delta_e=aero_data(5,4); Cm_delta_a=aero_data(5,5); Cm_delta_r=aero_data(5,6); Cm_p=aero_data(5,7);Cm_q=aero_data(5,8);Cm_r=aero_data(5,9);

Cno =aero_data(6,1); Cn_alpha=aero_data(6,2);Cn_beta=aero_data(6,3); Cn_delta_e=aero_data(6,4); Cn_delta_a=aero_data(6,5); Cn_delta_r=aero_data(6,6); Cn_p=aero_data(6,7);Cn_q=aero_data(6,8);Cn_r=aero_data(6,9);


% %% perturbation in Aero coffecients
% CLo =CLo*aero_coff_pert_factor(1,1); CL_alpha=CL_alpha*aero_coff_pert_factor(1,2);CL_beta=CL_beta*aero_coff_pert_factor(1,3); CL_delta_e=CL_delta_e*aero_coff_pert_factor(1,4); CL_delta_a=CL_delta_a*aero_coff_pert_factor(1,5); CL_delta_r=CL_delta_r*aero_coff_pert_factor(1,6); CL_p=CL_p*aero_coff_pert_factor(1,7);CL_q=CL_q*aero_coff_pert_factor(1,8);CL_r=CL_r*aero_coff_pert_factor(1,9);
% 
% Cdo =Cdo*aero_coff_pert_factor(2,1); Cd_alpha=Cd_alpha*aero_coff_pert_factor(2,2);Cd_beta=Cd_beta*aero_coff_pert_factor(2,3); Cd_delta_e=Cd_delta_e*aero_coff_pert_factor(2,4); Cd_delta_a=Cd_delta_a*aero_coff_pert_factor(2,5); Cd_delta_r=Cd_delta_r*aero_coff_pert_factor(2,6); Cd_p=Cd_p*aero_coff_pert_factor(2,7);Cd_q=Cd_q*aero_coff_pert_factor(2,8);Cd_r=Cd_r*aero_coff_pert_factor(2,9);
% 
% CYo =CYo*aero_coff_pert_factor(3,1); CY_alpha=CY_alpha*aero_coff_pert_factor(3,2);CY_beta=CY_beta*aero_coff_pert_factor(3,3); CY_delta_e=CY_delta_e*aero_coff_pert_factor(3,4); CY_delta_a=CY_delta_a*aero_coff_pert_factor(3,5); CY_delta_r=CY_delta_r*aero_coff_pert_factor(3,6); CY_p=CY_p*aero_coff_pert_factor(3,7);CY_q=CY_q*aero_coff_pert_factor(3,8);CY_r=CY_r*aero_coff_pert_factor(3,9);
% 
% Clo =Clo*aero_coff_pert_factor(4,1); Cl_alpha=Cl_alpha*aero_coff_pert_factor(4,2);Cl_beta=Cl_beta*aero_coff_pert_factor(4,3); Cl_delta_e=Cl_delta_e*aero_coff_pert_factor(4,4); Cl_delta_a=Cl_delta_a*aero_coff_pert_factor(4,5); Cl_delta_r=Cl_delta_r*aero_coff_pert_factor(4,6); Cl_p=Cl_p*aero_coff_pert_factor(4,7);Cl_q=Cl_q*aero_coff_pert_factor(4,8);Cl_r=Cl_r*aero_coff_pert_factor(4,9);
% 
% Cmo =Cmo*aero_coff_pert_factor(5,1); Cm_alpha=Cm_alpha*aero_coff_pert_factor(5,2);Cm_beta=Cm_beta*aero_coff_pert_factor(5,3); Cm_delta_e=Cm_delta_e*aero_coff_pert_factor(5,4); Cm_delta_a=Cm_delta_a*aero_coff_pert_factor(5,5); Cm_delta_r=Cm_delta_r*aero_coff_pert_factor(5,6); Cm_p=Cm_p*aero_coff_pert_factor(5,7);Cm_q=Cm_q*aero_coff_pert_factor(5,8);Cm_r=Cm_r*aero_coff_pert_factor(5,9);
% 
% Cno =Cno*aero_coff_pert_factor(6,1); Cn_alpha=Cn_alpha*aero_coff_pert_factor(6,2);Cn_beta=Cn_beta*aero_coff_pert_factor(6,3); Cn_delta_e=Cn_delta_e*aero_coff_pert_factor(6,4); Cn_delta_a=Cn_delta_a*aero_coff_pert_factor(6,5); Cn_delta_r=Cn_delta_r*aero_coff_pert_factor(6,6); Cn_p=Cn_p*aero_coff_pert_factor(6,7);Cn_q=Cn_q*aero_coff_pert_factor(6,8);Cn_r=Cn_r*aero_coff_pert_factor(6,9);
% %%

Cd_brake=0.0;brake=0.0;g=9.81;



u=Plane_state(1);
v=Plane_state(2);
w=Plane_state(3);
p=Plane_state(4);
q=Plane_state(5);
r=Plane_state(6);
phi=Plane_state(7);
theta=Plane_state(8);
psi=Plane_state(9);
X=Plane_state(10);
Y=Plane_state(11);
Z=Plane_state(12);



Tzf=Tzf2+Tzf3;
Tzb=Tzb6+Tzb7;
Tx=Tx9+Tx10;


R_v_v1=[cos(psi) sin(psi) 0; -sin(psi) cos(psi) 0; 0 0 1];
R_v1_v2=[cos(theta) 0 -sin(theta) ;0 1 0; sin(theta) 0 cos(theta)];
R_v2_b=[1 0 0;0 cos(phi) sin(phi) ;0 -sin(phi) cos(phi)];
R_v_b=R_v2_b*R_v1_v2*R_v_v1;


% 
% Wind_ned(1)=Wind_ned(1)*wind_pert_factor(1);% adding perturbation to wind components
% Wind_ned(2)=Wind_ned(2)*wind_pert_factor(2);
% Wind_ned(3)=Wind_ned(3)*wind_pert_factor(3);

V_wind_bd=R_v_b*[Wind_ned(1);Wind_ned(2);Wind_ned(3)];

ppp = [u-V_wind_bd(1); v; w];
u_r=ppp(1);
v_r=ppp(2);
w_r=ppp(3);

V=sqrt(u_r^2+v_r^2+w_r^2);


if (u_r^2+v_r^2+w_r^2)<=0.1
    alpha=0;
else
    alpha=atan2( w_r, u_r);
end


if norm(u_r) < 10^-1  && norm(v_r) < 10^-1 && norm(w_r) < 10^-1
    beta=0;
else
    beta = asin(v_r/sqrt(u_r^2+v_r^2+w_r^2));
end


R_b_s=[cos(alpha) 0 sin(alpha) ;0 1 0; -sin(alpha) 0 cos(alpha)];
R_s_w=[cos(beta) sin(beta) 0; -sin(beta) cos(beta) 0; 0 0 1];
R_w_b=(R_b_s)'*(R_s_w)';


u_dot_d=acc_d(1);
v_dot_d=acc_d(2);
w_dot_d=acc_d(3);

mg_b = R_v_b*[0 ;0; mass*g];
D=0.5*rho*V*V*s*(Cdo+Cd_alpha*abs(alpha)+Cd_delta_e*abs(delta_e)+ Cd_brake*abs(brake)) ;
D_b=R_w_b*[-D;0;0];

if V<0.1
    CL = CLo + CL_alpha*alpha + CL_delta_e*delta_e ;
else
    CL = CLo + CL_alpha*alpha + CL_delta_e*delta_e  + CL_q*q*c/(2*V) ;
end
L=0.5*rho*V*V*s*(CL);
L_b = R_w_b*[0;0;-L];
if abs(V)<0.1
    CY=CYo + CY_delta_r*delta_r + CY_beta*beta;
else
    CY=CYo + CY_delta_r*delta_r + CY_beta*beta + CY_r*r*b/(2*V);
end
FY=0.5*rho*V*V*s*(CY);

l_aero=0.5*rho*V^2*s*b*( Clo + Cl_delta_a*delta_a +Cl_delta_r*delta_r +Cl_beta*beta )+0.5*rho*V*s*b*(Cl_p*p*b/2+Cl_r*r*b/2);
m_aero=0.5*rho*V^2*s*c*( Cmo + Cm_alpha*alpha + Cm_delta_e*delta_e)+0.5*rho*V*s*c*Cm_q*q*c/2;
n_aero=0.5*rho*V^2*s*b*( Cno + Cn_delta_a*delta_a +Cn_delta_r*delta_r +Cn_beta*beta )+0.5*rho*V*s*b*(Cn_r*r*b/2+ Cn_p*p*b/2);


l=l_aero - Tzf2*y2*cos(mb) - Tzf3*y3*cos(mb)   - Tzb6*y6*cos(mb) - Tzb7*y7*cos(mb);
m=m_aero + Tzf*x1*cos(mb) + Tzb*x2*cos(mb) + Tx9*z9 + d1*Tzf2*b1_inv*sin(mb) - d1*Tzf3*b1_inv*sin(mb) - d1*Tzb6*b1_inv*sin(mb) + d1*Tzb7*b1_inv*sin(mb) ;
%	n=n_aero - Tx9_real*y9  - d1*Tzf2_real/b1 + d1*Tzf3_real/b1 + d1*Tzb6_real/b1 - d1*Tzb7_real/b1 ; //optimization
n=n_aero - Tx9*y9 - Tx10*y10 + (Tzf2*x1*sin(mb) - Tzf3*x1*sin(mb) +  Tzb6*x2*sin(mb) - Tzb7*x2*sin(mb)) - d1*Tzf2*b1_inv*cos(mb) + d1*Tzf3*b1_inv*cos(mb)  + d1*Tzb6*b1_inv*cos(mb)  - d1*Tzb7*b1_inv*cos(mb)  ;



fx = Tx9 + Tx10 + D_b(1)+ mg_b(1)+L_b(1);
%%%%%%%%%%%%%%%%%%%%%%%%%%%%%%%%%%%%%%%%%%%%%%%%%%%%%%%%%%%%%%%%%%%%%%%%%%%
fy = (Tzf2*sin(mb) - Tzf3*sin(mb) + Tzb6*sin(mb) - Tzb7*sin(mb)) + D_b(2) + mg_b(2) + FY + L_b(2);
%%%%%%%%%%%%%%%%%%%%%%%%%%%%%%%%%%%%%%%%%%%%%%%%%%%%%%%%%%%%%%%%%%%%%%%%%%%
fz = -Tzf*cos(mb) - Tzb*cos(mb) + mg_b(3)+D_b(3)+L_b(3);



tam=[-b1*y2,-b1*y3,-b1*y6,-b1*y7; b1*x1,b1*x1,b1*x2,b1*x2; -d1,d1,d1,-d1; -b1,-b1,-b1,-b1];
tbm=zeros(4,1);
tbm(1)=(((p_dot_d - c1*p*q + c2*(q*r) -c4*n)*c3_inv) - l_aero);%//(((p_dot_d - c1*p*q + c2*(q*r) -c4*n)/c3) - l_aero)*w1*3/8
tbm(2)=(((q_dot_d - c5*p*r + c6*(p*p-r*r))*Iy) - m_aero);%//(((q_dot_d - c5*p*r + c6*(p*p-r*r))*Iy) - m_aero)*w1/2
tbm(3)=(((r_dot_d - c7*p*q + c1*(q*r) -c4*l)*c8_inv) - n_aero);%//(((r_dot_d - c7*p*q + c1*(q*r) -c4*l)/c8) - n_aero)*w1/2
tbm(4)=(mass*w_dot_d - mg_b(3) - D_b(3) -L_b(3));%//(mass*w_dot_d - mg_b(3) - D_b(3) -L_b(3))/2
omega_velocity=inv(tam)*tbm;

for i=1:4
    if omega_velocity(i)<0.0
        omega_velocity(i)=0.0;
    end
end
omega_2=sqrt(omega_velocity(1));
omega_3=sqrt(omega_velocity(2));
omega_6=sqrt(omega_velocity(3));
omega_7=sqrt(omega_velocity(4));


Tzf2=b1*omega_2^2;

Tzf3=b1*omega_3^2;

Tzb6=b1*omega_6^2;

Tzb7=b1*omega_7^2;

Tzf=Tzf2+Tzf3;
Tzb=Tzb6+Tzb7;
Tx=Tx9+Tx10;

Tzf1=0.0;
Tzf4=0.0;
Tzb5=0.0;
Tzb8=0.0;
Tx9=0.0;
Tx10=0.0;
delta_e=0.0;
delta_a=0.0;
delta_r=0.0;

if(Tzf > (T_by_W*mass*g)/2.0)
    
    Tzf=(T_by_W*mass*g)/2.0;
end
if(Tzf<= 0.0)
    
    Tzf=0.0;
end

if(Tzf2<=0.0)
    
    Tzf2=0.0;
end
if(Tzf3<= 0.0)
    
    Tzf3=0.0;
end

if(Tzb> (T_by_W*mass*g)/2.0)
    
    Tzb=(T_by_W*mass*g)/2.0;
end



if(Tzb6<= 0.0)
    
    Tzb6=0.0;
end
if(Tzb7<=0.0)
    
    Tzb7=0.0;
end

if(Tzb<= 0.0)
    
    Tzb=0.0;
end

if(Tx< 0.0)
    
    Tx=0.0;
end

if(Tx9 < 0.0)
    
    Tx9=0.0;
end


if(Tx>60.0)
    
    Tx=60.0;
end

if((Tx9)>60.0)
    
    Tx9=60.0;
end

if(Tx10 < 0.0)
    
    Tx10=0.0;
end

if(Tzf2>(T_by_W*mass*g)/4.0)
    
    Tzf2 =(T_by_W*mass*g)/4.0;
end
if(Tzf3>=(T_by_W*mass*g)/4.0)
    
    Tzf3 =(T_by_W*mass*g)/4.0;
end

if(Tzb6>=(T_by_W*mass*g)/4.0)
    
    Tzb6 =(T_by_W*mass*g)/4.0;
end
if(Tzb7>=(T_by_W*mass*g)/4.0)
    
    Tzb7 =(T_by_W*mass*g)/4.0;
end

end
